simulink model "Adding_Noise"  (R2018a)
settings: Solver=VariableStepAuto  StartTime=0.0  StopTime=10.0  RelTol=1e-3
settings Model: Creator=ashwin  LastModifiedBy=ashwin

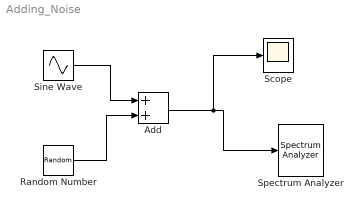
== system Adding_Noise ==
  "Add " : Sum
  "Random Number " : RandomNumber  Variance=0.1  SampleTime=0.001
  "Scope " : Scope
  "Sine Wave " : Sin  Frequency=2*pi*50  SampleTime=0.001
  "Spectrum Analyzer " : SpectrumAnalyzer
  wires:
  "Random Number "/1 -> "Add "/2
  "Sine Wave "/1 -> "Add "/1
  "Add "/1 -> "Scope "/1, "Spectrum Analyzer "/1
